simulink model "prescan_repl_getObjectObserversCarObserver"  (R2019a)
settings: Solver=VariableStepAuto  StartTime=0.0  StopTime=100  RelTol=1e-3
libraries: ProSivic_Sensors x2, realtime_pacer_lib x1
settings Model: Creator=Markus Borg  LastModifiedBy=Markus Borg

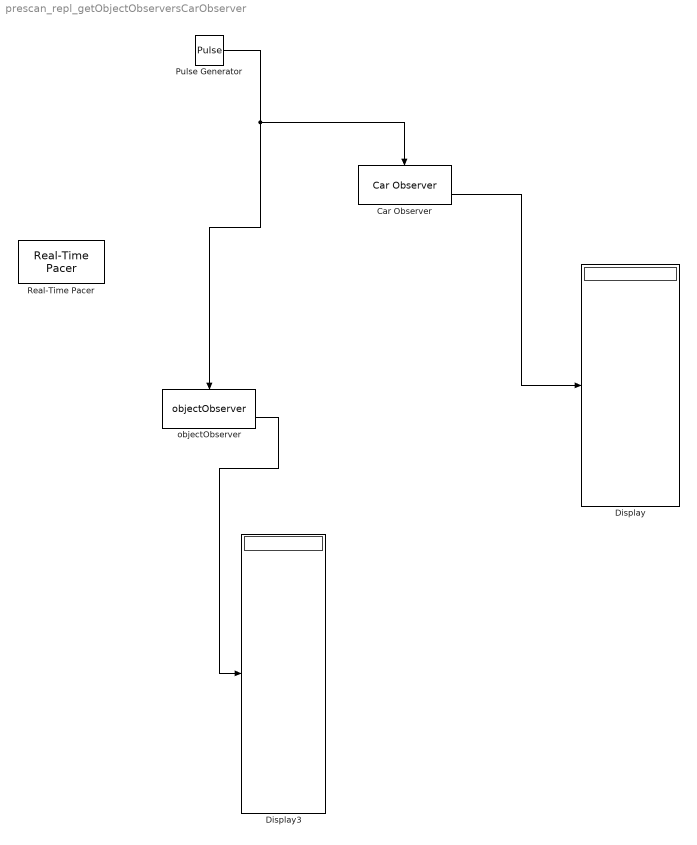
== system prescan_repl_getObjectObserversCarObserver ==
  Car Observer : ProSivic_Sensors/Car Observer  SystemSampleTime=-1
      link override S-Function: topic=egocar_obs
  Display : Display
  Display3 : Display
  Pulse Generator : DiscretePulseGenerator  PulseType=Time based  Period=0.5  PulseWidth=50
  Real-Time Pacer : realtime_pacer_lib/Real-Time Pacer  simTimePerRealTime=10
  objectObserver : ProSivic_Sensors/objectObserver  topic=ped_obs
  wires:
  Pulse Generator/1 -> Car Observer/Trigger, objectObserver/Trigger
  objectObserver/2 -> Display3/1
  Car Observer/2 -> Display/1
